simulink model "Problem_2"  (R2020a)
settings: Solver=VariableStepAuto  StartTime=0.0  StopTime=100  RelTol=1e-3
undefined symbols (not defined in the file): b, k1, K2, m1, m2
settings Model: Creator=Admin  LastModifiedBy=Admin
settings DataIOCC: ExternalInput=[t,stin]  LoadExternalInput=on  SaveFormat=Array

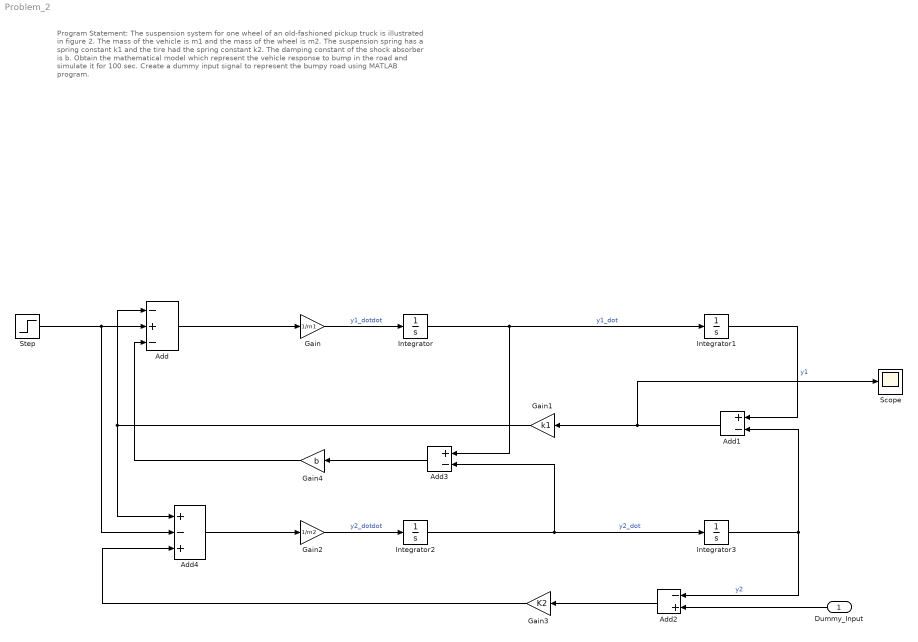
== system Problem_2 ==
  note: Program Statement:
      | The suspension system for one wheel of an old-fashioned pickup truck is illustrated in figure 2.
      | The mass of the vehicle is m1 and the mass of the wheel is m2. The suspension spring has a
      | spring constant k1 and the tire had the spring constant k2. The damping constant of the shock
      | absorber is b. Obtain the mathematical model which represent the vehicle response to bump in
      | the road and simulate it for 100 sec. Create a dummy input signal to represent the bumpy road using MATLAB program.
  Dummy_Input : Inport
  Add : Sum  Inputs=-+-
  Add1 : Sum  Inputs=+-
  Add2 : Sum  Inputs=-+
  Add3 : Sum  Inputs=+-
  Add4 : Sum  Inputs=+-+
  Gain : Gain  Gain=1/m1
  Gain1 : Gain  Gain=k1
  Gain2 : Gain  Gain=1/m2
  Gain3 : Gain  Gain=K2
  Gain4 : Gain  Gain=b
  Integrator{,1..3} (4 alike) : Integrator
  Scope : Scope
  Step : Step  SampleTime=0
  wires:
  Integrator/1 -> Add3/1, Integrator1/1  "y1_dot"
  Gain/1 -> Integrator/1  "y1_dotdot"
  Add/1 -> Gain/1
  Add1/1 -> Scope/1, Gain1/1
  Integrator1/1 -> Add1/1  "y1"
  Integrator3/1 -> Add2/1, Add1/2  "y2"
  Add2/1 -> Gain3/1
  Integrator2/1 -> Add3/2, Integrator3/1  "y2_dot"
  Add3/1 -> Gain4/1
  Gain2/1 -> Integrator2/1  "y2_dotdot"
  Add4/1 -> Gain2/1
  Gain3/1 -> Add4/3
  Step/1 -> Add/2, Add4/2
  Gain4/1 -> Add/3
  Gain1/1 -> Add4/1, Add/1
  Dummy_Input/1 -> Add2/2
